simulink model "sim_punto_3"  (R2021b)
settings: Solver=VariableStepAuto  StartTime=0.0  StopTime=50  RelTol=1e-3
values from neighbouring files (symbols this model uses):
  A = [0 1 0 0 0 0 0 0 0 0 0 0 ... (first row only)    [punto3.m]
  B = [0; 0; 0; 0; 0; 0; 0; 0; 0; 0; 0; 1]    [punto3.m]
  C = [1 0 0 0 0 0 0 0 0 0 0 0]    [punto3.m]
  C_states = eye(12)    [punto3.m]
  D_states = [0 0 0 0 0 0 0 0 0 0 0 0]'    [punto3.m]
  N1 = 3    [punto3.m]
  N2 = 6    [punto3.m]
  N3 = 6    [punto3.m]
  Q = [1+q 0 0 0 0 0 0 0 0 0 0 0 ... (first row only)    [punto3.m]
  R = r    (= 1e-05)    [punto3.m]
  S = [0 0 0 0 0 0 0 0 0 0 0 0 ... (first row only)    [punto3.m]
  Ts = 0.1    [punto3.m]
  U_max = 15    [punto3.m]
  U_min = -15    [punto3.m]
  Ubar = inv(g)*Ybar    [punto3.m]
  x0 = [0 0 0 0 0 0 0 0 0 0 0 0]'    [punto3.m]
  Xbar = -inv(A) * B * Ubar    [punto3.m]
undefined symbols (not defined in the file or in its folder): mympc
settings Model: Creator=danie  LastModifiedBy=danie

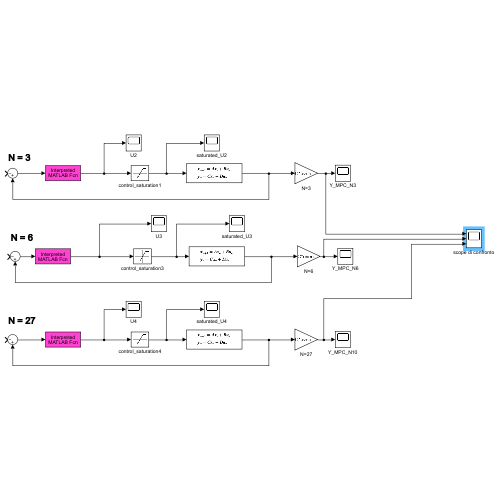
[thumbnail: Simulink's stored preview of the top-level diagram]
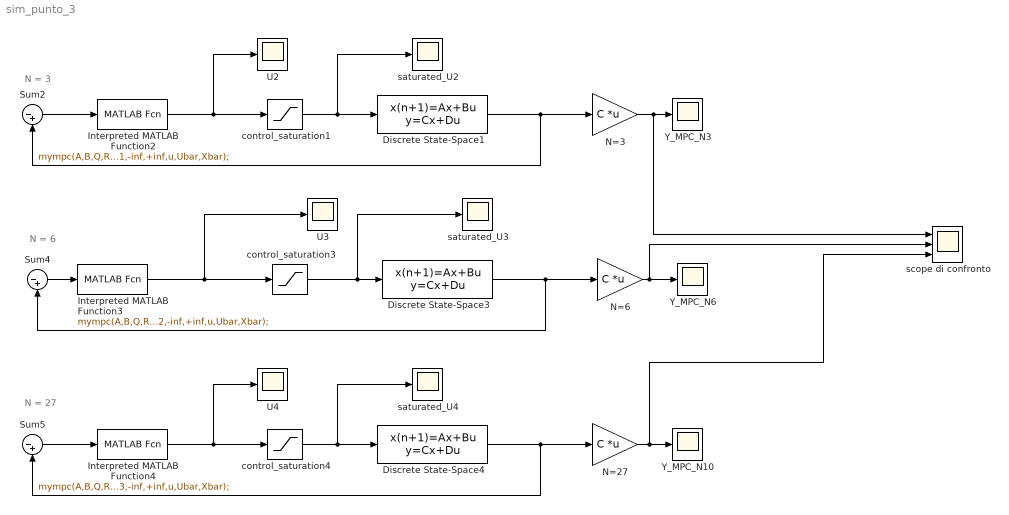
== system sim_punto_3 ==
  note: N = 3
  note: N = 6
  note: N = 27
  Discrete State-Space1 : DiscreteStateSpace  A=A  B=B  C=C_states  D=D_states  InitialCondition=x0  SampleTime=Ts
  Discrete State-Space3 : DiscreteStateSpace  A=A  B=B  C=C_states  D=D_states  InitialCondition=x0  SampleTime=Ts
  Discrete State-Space4 : DiscreteStateSpace  A=A  B=B  C=C_states  D=D_states  InitialCondition=x0  SampleTime=Ts
  Interpreted MATLAB Function2 : MATLABFcn  MATLABFcn=mympc(A,B,Q,R,S,N1,-inf,+inf,u,Ubar,Xbar);  OutputDimensions=1
  Interpreted MATLAB Function3 : MATLABFcn  MATLABFcn=mympc(A,B,Q,R,S,N2,-inf,+inf,u,Ubar,Xbar);  OutputDimensions=1
  Interpreted MATLAB Function4 : MATLABFcn  MATLABFcn=mympc(A,B,Q,R,S,N3,-inf,+inf,u,Ubar,Xbar);  OutputDimensions=1
  N=27 : Gain  Gain=C  Multiplication=Matrix(K*u) (u vector)
  N=3 : Gain  Gain=C  Multiplication=Matrix(K*u) (u vector)
  N=6 : Gain  Gain=C  Multiplication=Matrix(K*u) (u vector)
  Sum2 : Sum  Inputs=|-+
  Sum4 : Sum  Inputs=|-+
  Sum5 : Sum  Inputs=|-+
  U2 : Scope
  U3 : Scope
  U4 : Scope
  Y_MPC_N10 : Scope
  Y_MPC_N3 : Scope
  Y_MPC_N6 : Scope
  control_saturation1 : Saturate  UpperLimit=U_max  LowerLimit=U_min
  control_saturation3 : Saturate  UpperLimit=inf  LowerLimit=-inf
  control_saturation4 : Saturate  UpperLimit=inf  LowerLimit=-inf
  saturated_U2 : Scope
  saturated_U3 : Scope
  saturated_U4 : Scope
  scope di confronto : Scope  NumInputPorts=3
  wires:
  N=27/1 -> scope di confronto/3, Y_MPC_N10/1
  Interpreted MATLAB Function4/1 -> control_saturation4/1, U4/1
  Discrete State-Space4/1 -> Sum5/2, N=27/1
  control_saturation4/1 -> saturated_U4/1, Discrete State-Space4/1
  Discrete State-Space1/1 -> Sum2/2, N=3/1
  Discrete State-Space3/1 -> Sum4/2, N=6/1
  Sum4/1 -> Interpreted MATLAB Function3/1
  N=6/1 -> scope di confronto/2, Y_MPC_N6/1
  Interpreted MATLAB Function2/1 -> control_saturation1/1, U2/1
  N=3/1 -> scope di confronto/1, Y_MPC_N3/1
  control_saturation3/1 -> saturated_U3/1, Discrete State-Space3/1
  control_saturation1/1 -> saturated_U2/1, Discrete State-Space1/1
  Sum5/1 -> Interpreted MATLAB Function4/1
  Interpreted MATLAB Function3/1 -> control_saturation3/1, U3/1
  Sum2/1 -> Interpreted MATLAB Function2/1
